simulink model "solarproject"  (R2023b)
settings: Solver=ode23t  StartTime=0.0  StopTime=1  RelTol=1e-3
undefined symbols (not defined in the file): Acid, Lead
libraries: spsSeriesRLCBranchLib x3, spsBatteryLib x1, spsDiodeLib x1, simulink x1, spsMosfetLib x1, spsPVArrayLib x1, sps_lib x1
settings Model: Creator=oiaon  LastModifiedBy=oiaon

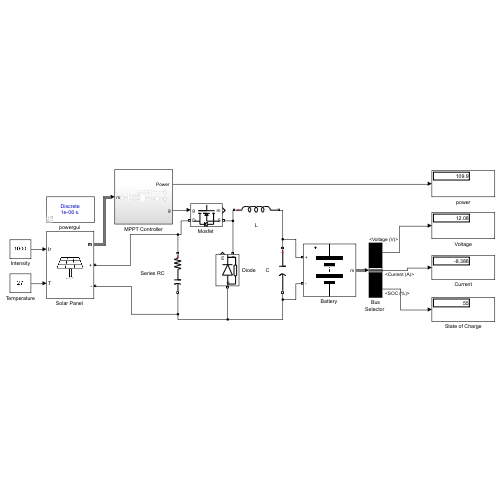
[thumbnail: Simulink's stored preview of the top-level diagram]
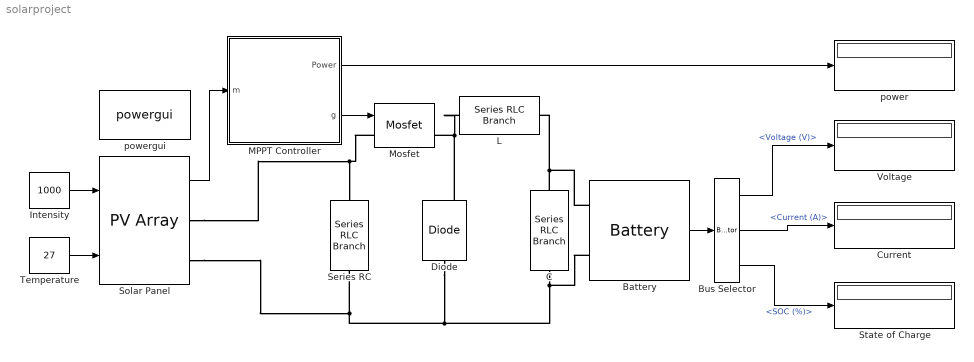
== system solarproject ==
  "Battery " : spsBatteryLib/Battery  BatType=Lead-Acid  ShowTempParam=off  ThermalPreset=no  ShowAgeParam=off  NomV=12  NomQ=100  SOC=55  Batt_Tr=1  PresetModel=on  MaxQ=104.1667  MinV=9  FullV=13.0658  Dis_rate=20  R=0.0012  Normal_OP=31.0278  expZone="[12.2171     0.333333]"  current=[6.5 13 32.5]  Units=Time  Tci=20  NomT=20  T2=-30  MaxQ2=4.8  FullV2=7.1  Normal_OP2=5.655  expZone2="[6.58           1]"  Rca=0.6  ti=2000  Dp=0  Neq0=0  Tsim=1e6  Ta1=25  Qeol=5.4*0.9  Reol=0.013333*1.2  Char_age=[2.3478, 3]  Dis_age=[2.3478, 10]  N1=1500  N2=10500  N3=1000  N4=1400  Ta2=45  N5=950
  "Bus Selector " : BusSelector  OutputSignals=Voltage (V),Current (A),SOC (%)
  C : spsSeriesRLCBranchLib/Series RLC Branch  LConnTagsString=__new0  RConnTagsString=__new0  BranchType=C  Resistance=1  Inductance=0.783e-3  SetiL0=off  InitialCurrent=0  Capacitance=364e-6  Setx0=off  InitialVoltage=0  Measurements=None
  Current : Display
  "Diode " : spsDiodeLib/Diode  Ron=0.001  Lon=0  Vf=0.8  IC=0  UseSnubber=0  Rs=500  Cs=250e-9  Measurements=on
  Intensity : Constant  Value=1000
  L : spsSeriesRLCBranchLib/Series RLC Branch  LConnTagsString=__new0  RConnTagsString=__new0  BranchType=L  Resistance=1  Inductance=0.783e-3  SetiL0=off  InitialCurrent=0  Capacitance=1e-6  Setx0=off  InitialVoltage=0  Measurements=None
  MPPT Controller : Subsystem
  "Mosfet " : spsMosfetLib/Mosfet  Ron=0.1  Lon=0  Rd=0.01  Vfd=0  IC=0  Rs=1e5  Cs=inf  Measurements=on
  Series RC : spsSeriesRLCBranchLib/Series RLC Branch  LConnTagsString=__new0  RConnTagsString=__new0  BranchType=RC  Resistance=0.0001  Inductance=1e-3  SetiL0=off  InitialCurrent=0  Capacitance=1000e-6  Setx0=off  InitialVoltage=0  Measurements=None
  "Solar Panel " : spsPVArrayLib/PV Array  Npar=1  Nser=1  PlotType=array @ 1000 W/m2 & specified temperatures  S_vec="[ 1000  500  100 ]"  Temp_C_vec="[ 45 25  ]"  ModuleName=User-defined  PlotWhenSelected=off  Pm=213.15  Ncell=60  Voc=36.3  Isc=7.84  Vm=29  Im=7.35  beta_Voc_pc=-0.36099  alpha_Isc_pc=0.102  beta_Voc=-0.13104  alpha_Isc=0.0079968  IL=7.8654  I0=2.9273e-10  nI=0.98119  Rsh=313.0553  Rs=0.39381  RobustModel=off  RobustCellTemperature=313.3991  BAL=on  Tc=1e-6  Tfilter=5e-5
  State of Charge : Display
  Temperature : Constant  Value=27
  Voltage : Display
  power : Display
  "powergui " : sps_lib/powergui  Priority=1  SimulationMode=Discrete  SampleTime=1e-6  frequency=60  Iterations=50  frequencyindice=0  Pbase=100e6  ErrMax=1e-4  UnitsV=kV  UnitsW=MW  buscounter=0  FunctionMessages=off  echomessages=off  EnableUseOfTLC=off  CurrentSourceSwitches=off  DisableSnubberDevices=off  DisableRonSwitches=off  DisableVfSwitches=off  DisplayEquations=off  AutomaticDiscreteSolvers=off  SolverType=Tustin/Backward Euler (TBE)  Interpol=off  ExternalGateDelay=off  methode=off  Ts=100  x0status=blocks  SPID=on  SwTol=0  HookPort=off  NonlinearTolerance=1e-4  nMaxIteration=100  ContinueOnMaxIteration=off  RestoreLinks=warning  ResistiveCurrentMeasurement=off  Frange=[0:2:500]  Ylog=off  Xlog=on  ShowGrid=off  save=off  variable=ZData  structure=0  ZoomFFT=off  StartTime=0.0  cycles=1  DisplayStyle=1  fundamental=60  FreqAxis=off  MaxFrequency=1000  frequencyindicesteady=1  RmsSteady=1  display=off
  wires:
  "Solar Panel "/1 -> MPPT Controller/1(m)
  Temperature/1 -> "Solar Panel "/2
  "Bus Selector "/2 -> Current/1  "<Current (A)>"
  "Battery "/1 -> "Bus Selector "/1
  "Bus Selector "/1 -> Voltage/1  "<Voltage (V)>"
  "Bus Selector "/3 -> State of Charge/1  "<SOC (%)>"
  Intensity/1 -> "Solar Panel "/1
  MPPT Controller/1("Power ") -> power/1
  MPPT Controller/2(g) -> "Mosfet "/1
  connections:
  "Diode "/RConn1 -- L/LConn1 -- "Mosfet "/RConn1
  "Mosfet "/LConn1 -- "Solar Panel "/RConn1 -- Series RC/LConn1
  C/RConn1 -- "Battery "/LConn2 -- Series RC/RConn1 -- "Solar Panel "/RConn2 -- "Diode "/LConn1
  C/LConn1 -- L/RConn1 -- "Battery "/LConn1

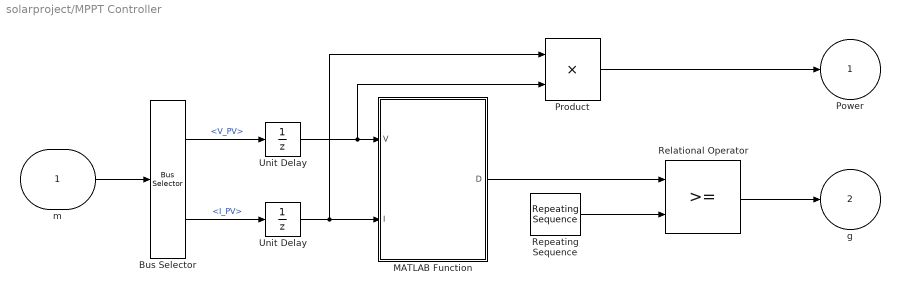
== system solarproject/MPPT Controller ==
  m : Inport
  "Bus Selector  " : BusSelector  OutputSignals=V_PV,I_PV
  "MATLAB Function " : MATLAB Function  TreatAsAtomicUnit=on
  "Product " : Product
  "Relational Operator " : RelationalOperator  OutDataTypeStr=boolean  RndMeth=Simplest  InputSameDT=off
  "Repeating Sequence " : simulink/Sources/Repeating Sequence  rep_seq_t=[0 0.0002]  rep_seq_y=[0 1]
  "Unit Delay " : UnitDelay  SampleTime=1e-4  HasFrameUpgradeWarning=on
  "Unit Delay  " : UnitDelay  SampleTime=1e-4  HasFrameUpgradeWarning=on
  "Power " : Outport
  g : Outport  Port=2
  wires:
  m/1 -> "Bus Selector  "/1
  "Unit Delay "/1 -> "Product "/2, "MATLAB Function "/1(V)
  "Relational Operator "/1 -> g/1
  "Repeating Sequence "/1 -> "Relational Operator "/2
  "MATLAB Function "/1(D) -> "Relational Operator "/1
  "Unit Delay  "/1 -> "Product "/1, "MATLAB Function "/2(I)
  "Product "/1 -> "Power "/1
  "Bus Selector  "/1 -> "Unit Delay "/1  "<V_PV>"
  "Bus Selector  "/2 -> "Unit Delay  "/1  "<I_PV>"

== matlab function solarproject/MPPT Controller/MATLAB Function  ==
  data: V input; D output; I input
function D = DutyRatio (V, I)
Dmax =0.95;
Dmin=0;
Dinit =0.95;
deltaD=0.001;
persistent Vold Pold Dold;
dataType = 'double';

if isempty(Vold)
    Vold=0;
    Pold=0;
    Dold = Dinit;
end
P=V*I;
dV= V-Vold;
dP= P-Pold;

if dP ~= 0
    if dP<0
        if dV<0
           D= Dold - deltaD;
        else
           D= Dold + deltaD;
        end
    else
        if  dV<0
            D= Dold + deltaD;
        else
            D= Dold - deltaD;
        end
    end
else D= Dold;
end   
if D>= Dmax | D<= Dmin
    D=Dold;
end
Dold= D;
VOld= V;
Pold= P;
